simulink model "end_sem_mimuro_plot"  (R2023b)
settings: Solver=FixedStepAuto  StartTime=0.0  StopTime=20  FixedStep=0.001  RelTol=1e-3
undefined symbols (not defined in the file): simscape, X, Y, Z
libraries: sm_lib x108, nesl_utility x77, fl_lib x23, sdl_lib x5, sharedtransform x4
(part 6 of 6)

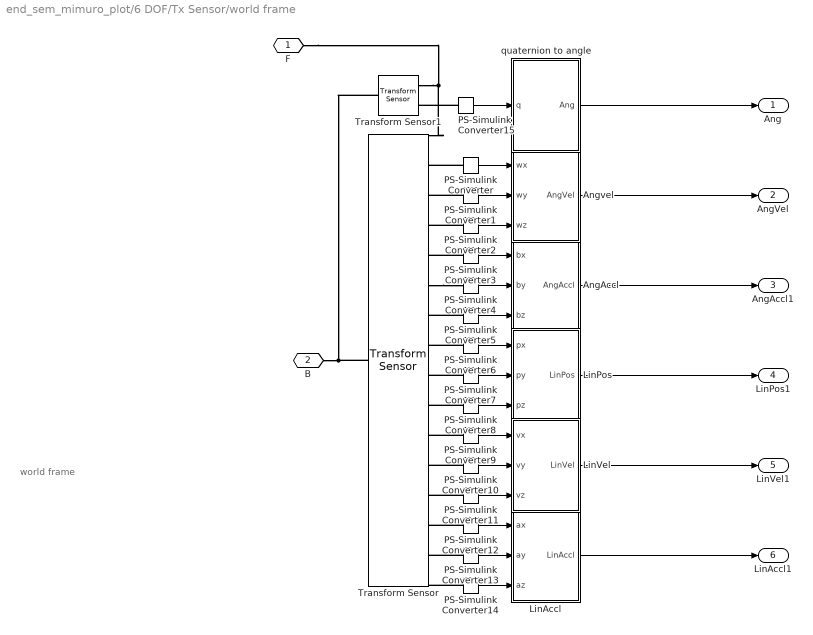
== system end_sem_mimuro_plot/6 DOF/Tx Sensor/world frame ==
  note: world frame
  AngAccl : Subsystem
  Angvel : Subsystem
  LinAccl : Subsystem
  LinPos : Subsystem
  LinVel : Subsystem
  PS-Simulink Converter{,1..15} (16 alike) : nesl_utility/PS-Simulink Converter  PhysicalDomain=network_engine_domain  SubClassName=ps_output  LeftPortType=input  RightPortType=output  PseudoPeriodic=off  Frequencies=[]  VectorFormat=1-D array  Unit=inherit  AffineConversion=off
  Transform Sensor1 : sm_lib/Frames and Transforms/Transform Sensor  MeasurementFrame=World  RotationSequence=XYX  SenseAngle=off  SenseAxis=off  SenseQ=on  SenseR=off  SenseRotationSequence=off  SenseOmegaX=off  SenseOmegaY=off  SenseOmegaZ=off  SenseOmega=off  SenseQDot=off  SenseRDot=off  SenseRotationSequenceDot=off  SenseAlphaX=off  SenseAlphaY=off  SenseAlphaZ=off  SenseAlpha=off  SenseQDDot=off  SenseRDDot=off  SenseX=off  SenseY=off  SenseZ=off  SenseXYZ=off  SenseRad=off  SenseAzim=off  SenseDist=off  SenseInc=off  SenseXDot=off  SenseYDot=off  SenseZDot=off  SenseXYZDot=off  SenseRadDot=off  SenseAzimDot=off  SenseDistDot=off  SenseIncDot=off  SenseXDDot=off  SenseYDDot=off  SenseZDDot=off  SenseXYZDDot=off  SenseRadDDot=off  SenseAzimDDot=off  SenseDistDDot=off  SenseIncDDot=off
  Transform Sensor : sm_lib/Frames and Transforms/Transform Sensor  MeasurementFrame=World  RotationSequence=XYX  SenseAngle=off  SenseAxis=off  SenseQ=off  SenseR=off  SenseRotationSequence=off  SenseOmegaX=on  SenseOmegaY=on  SenseOmegaZ=on  SenseOmega=off  SenseQDot=off  SenseRDot=off  SenseRotationSequenceDot=off  SenseAlphaX=on  SenseAlphaY=on  SenseAlphaZ=on  SenseAlpha=off  SenseQDDot=off  SenseRDDot=off  SenseX=on  SenseY=on  SenseZ=on  SenseXYZ=off  SenseRad=off  SenseAzim=off  SenseDist=off  SenseInc=off  SenseXDot=on  SenseYDot=on  SenseZDot=on  SenseXYZDot=off  SenseRadDot=off  SenseAzimDot=off  SenseDistDot=off  SenseIncDot=off  SenseXDDot=on  SenseYDDot=on  SenseZDDot=on  SenseXYZDDot=off  SenseRadDDot=off  SenseAzimDDot=off  SenseDistDDot=off  SenseIncDDot=off
  quaternion to angle : Subsystem
  F : PMIOPort  Side=Left
  B : PMIOPort  Port=2  Side=Left
  Ang : Outport
  AngVel : Outport  Port=2
  AngAccl1 : Outport  Port=3
  LinPos1 : Outport  Port=4
  LinVel1 : Outport  Port=5
  LinAccl1 : Outport  Port=6
  wires:
  PS-Simulink Converter6/1 -> LinPos/1(px)
  PS-Simulink Converter4/1 -> AngAccl/2(by)
  PS-Simulink Converter14/1 -> LinAccl/3(az)
  PS-Simulink Converter10/1 -> LinVel/2(vy)
  PS-Simulink Converter3/1 -> AngAccl/1(bx)
  PS-Simulink Converter11/1 -> LinVel/3(vz)
  PS-Simulink Converter2/1 -> Angvel/3(wz)
  PS-Simulink Converter9/1 -> LinVel/1(vx)
  PS-Simulink Converter12/1 -> LinAccl/1(ax)
  PS-Simulink Converter13/1 -> LinAccl/2(ay)
  PS-Simulink Converter8/1 -> LinPos/3(pz)
  PS-Simulink Converter1/1 -> Angvel/2(wy)
  LinVel/1(LinVel) -> LinVel1/1
  PS-Simulink Converter/1 -> Angvel/1(wx)
  PS-Simulink Converter5/1 -> AngAccl/3(bz)
  PS-Simulink Converter15/1 -> quaternion to angle/1(q)
  PS-Simulink Converter7/1 -> LinPos/2(py)
  LinPos/1(LinPos) -> LinPos1/1
  LinAccl/1(LinAccl) -> LinAccl1/1
  AngAccl/1(AngAccl) -> AngAccl1/1
  Angvel/1(AngVel) -> AngVel/1
  quaternion to angle/1(Ang) -> Ang/1
  connections:
  Transform Sensor1/RConn1 -- Transform Sensor/RConn1 -- F/RConn1
  PS-Simulink Converter/LConn1 -- Transform Sensor/RConn2
  PS-Simulink Converter1/LConn1 -- Transform Sensor/RConn3
  PS-Simulink Converter12/LConn1 -- Transform Sensor/RConn14
  PS-Simulink Converter3/LConn1 -- Transform Sensor/RConn5
  PS-Simulink Converter2/LConn1 -- Transform Sensor/RConn4
  PS-Simulink Converter14/LConn1 -- Transform Sensor/RConn16
  PS-Simulink Converter7/LConn1 -- Transform Sensor/RConn9
  Transform Sensor/RConn6 -- PS-Simulink Converter4/LConn1
  PS-Simulink Converter5/LConn1 -- Transform Sensor/RConn7
  PS-Simulink Converter8/LConn1 -- Transform Sensor/RConn10
  PS-Simulink Converter6/LConn1 -- Transform Sensor/RConn8
  PS-Simulink Converter15/LConn1 -- Transform Sensor1/RConn2
  PS-Simulink Converter9/LConn1 -- Transform Sensor/RConn11
  PS-Simulink Converter13/LConn1 -- Transform Sensor/RConn15
  PS-Simulink Converter10/LConn1 -- Transform Sensor/RConn12
  PS-Simulink Converter11/LConn1 -- Transform Sensor/RConn13
  B/RConn1 -- Transform Sensor/LConn1 -- Transform Sensor1/LConn1

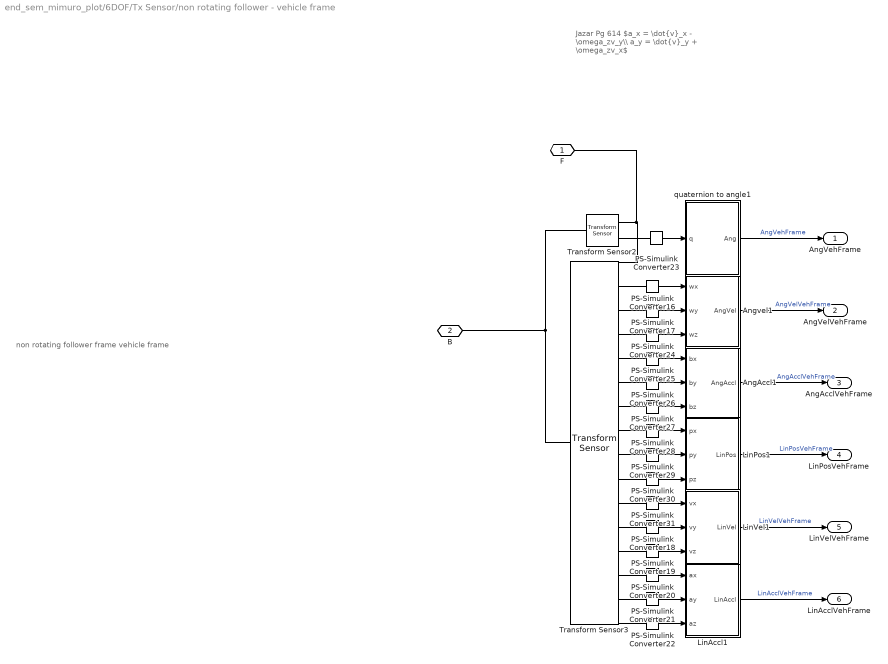
== system end_sem_mimuro_plot/6DOF/Tx Sensor/non rotating follower - vehicle frame ==
  note: non rotating follower frame
      | vehicle frame
  note: Jazar Pg 614
      | $a_x = \dot{v}_x - \omega_zv_y\\ a_y = \dot{v}_y + \omega_zv_x$
  AngAccl1 : Subsystem
  Angvel1 : Subsystem
  LinAccl1 : Subsystem
  LinPos1 : Subsystem
  LinVel1 : Subsystem
  PS-Simulink Converter{16..31} (16 alike) : nesl_utility/PS-Simulink Converter  PhysicalDomain=network_engine_domain  SubClassName=ps_output  LeftPortType=input  RightPortType=output  PseudoPeriodic=off  Frequencies=[]  VectorFormat=1-D array  Unit=inherit  AffineConversion=off
  Transform Sensor2 : sm_lib/Frames and Transforms/Transform Sensor  MeasurementFrame=NonRotatingFollower  RotationSequence=XYX  SenseAngle=off  SenseAxis=off  SenseQ=on  SenseR=off  SenseRotationSequence=off  SenseOmegaX=off  SenseOmegaY=off  SenseOmegaZ=off  SenseOmega=off  SenseQDot=off  SenseRDot=off  SenseRotationSequenceDot=off  SenseAlphaX=off  SenseAlphaY=off  SenseAlphaZ=off  SenseAlpha=off  SenseQDDot=off  SenseRDDot=off  SenseX=off  SenseY=off  SenseZ=off  SenseXYZ=off  SenseRad=off  SenseAzim=off  SenseDist=off  SenseInc=off  SenseXDot=off  SenseYDot=off  SenseZDot=off  SenseXYZDot=off  SenseRadDot=off  SenseAzimDot=off  SenseDistDot=off  SenseIncDot=off  SenseXDDot=off  SenseYDDot=off  SenseZDDot=off  SenseXYZDDot=off  SenseRadDDot=off  SenseAzimDDot=off  SenseDistDDot=off  SenseIncDDot=off
  Transform Sensor3 : sm_lib/Frames and Transforms/Transform Sensor  MeasurementFrame=NonRotatingFollower  RotationSequence=XYX  SenseAngle=off  SenseAxis=off  SenseQ=off  SenseR=off  SenseRotationSequence=off  SenseOmegaX=on  SenseOmegaY=on  SenseOmegaZ=on  SenseOmega=off  SenseQDot=off  SenseRDot=off  SenseRotationSequenceDot=off  SenseAlphaX=on  SenseAlphaY=on  SenseAlphaZ=on  SenseAlpha=off  SenseQDDot=off  SenseRDDot=off  SenseX=on  SenseY=on  SenseZ=on  SenseXYZ=off  SenseRad=off  SenseAzim=off  SenseDist=off  SenseInc=off  SenseXDot=on  SenseYDot=on  SenseZDot=on  SenseXYZDot=off  SenseRadDot=off  SenseAzimDot=off  SenseDistDot=off  SenseIncDot=off  SenseXDDot=on  SenseYDDot=on  SenseZDDot=on  SenseXYZDDot=off  SenseRadDDot=off  SenseAzimDDot=off  SenseDistDDot=off  SenseIncDDot=off
  quaternion to angle1 : Subsystem
  F : PMIOPort  Side=Left
  B : PMIOPort  Port=2  Side=Left
  AngVehFrame : Outport
  AngVelVehFrame : Outport  Port=2
  AngAcclVehFrame : Outport  Port=3
  LinPosVehFrame : Outport  Port=4
  LinVelVehFrame : Outport  Port=5
  LinAcclVehFrame : Outport  Port=6
  wires:
  PS-Simulink Converter16/1 -> Angvel1/1(wx)
  PS-Simulink Converter25/1 -> AngAccl1/1(bx)
  PS-Simulink Converter27/1 -> AngAccl1/3(bz)
  PS-Simulink Converter19/1 -> LinVel1/3(vz)
  quaternion to angle1/1(Ang) -> AngVehFrame/1  "AngVehFrame"
  PS-Simulink Converter20/1 -> LinAccl1/1(ax)
  Angvel1/1(AngVel) -> AngVelVehFrame/1  "AngVelVehFrame"
  PS-Simulink Converter31/1 -> LinVel1/1(vx)
  PS-Simulink Converter28/1 -> LinPos1/1(px)
  PS-Simulink Converter18/1 -> LinVel1/2(vy)
  PS-Simulink Converter30/1 -> LinPos1/3(pz)
  PS-Simulink Converter21/1 -> LinAccl1/2(ay)
  PS-Simulink Converter23/1 -> quaternion to angle1/1(q)
  PS-Simulink Converter22/1 -> LinAccl1/3(az)
  PS-Simulink Converter17/1 -> Angvel1/2(wy)
  PS-Simulink Converter24/1 -> Angvel1/3(wz)
  PS-Simulink Converter26/1 -> AngAccl1/2(by)
  PS-Simulink Converter29/1 -> LinPos1/2(py)
  LinVel1/1(LinVel) -> LinVelVehFrame/1  "LinVelVehFrame"
  AngAccl1/1(AngAccl) -> AngAcclVehFrame/1  "AngAcclVehFrame"
  LinPos1/1(LinPos) -> LinPosVehFrame/1  "LinPosVehFrame"
  LinAccl1/1(LinAccl) -> LinAcclVehFrame/1  "LinAcclVehFrame"
  connections:
  PS-Simulink Converter30/LConn1 -- Transform Sensor3/RConn10
  PS-Simulink Converter25/LConn1 -- Transform Sensor3/RConn5
  PS-Simulink Converter23/LConn1 -- Transform Sensor2/RConn2
  PS-Simulink Converter31/LConn1 -- Transform Sensor3/RConn11
  Transform Sensor2/LConn1 -- Transform Sensor3/LConn1 -- B/RConn1
  PS-Simulink Converter20/LConn1 -- Transform Sensor3/RConn14
  Transform Sensor2/RConn1 -- F/RConn1 -- Transform Sensor3/RConn1
  PS-Simulink Converter21/LConn1 -- Transform Sensor3/RConn15
  PS-Simulink Converter24/LConn1 -- Transform Sensor3/RConn4
  PS-Simulink Converter29/LConn1 -- Transform Sensor3/RConn9
  PS-Simulink Converter22/LConn1 -- Transform Sensor3/RConn16
  PS-Simulink Converter27/LConn1 -- Transform Sensor3/RConn7
  PS-Simulink Converter18/LConn1 -- Transform Sensor3/RConn12
  PS-Simulink Converter28/LConn1 -- Transform Sensor3/RConn8
  PS-Simulink Converter19/LConn1 -- Transform Sensor3/RConn13
  PS-Simulink Converter17/LConn1 -- Transform Sensor3/RConn3
  Transform Sensor3/RConn6 -- PS-Simulink Converter26/LConn1
  PS-Simulink Converter16/LConn1 -- Transform Sensor3/RConn2

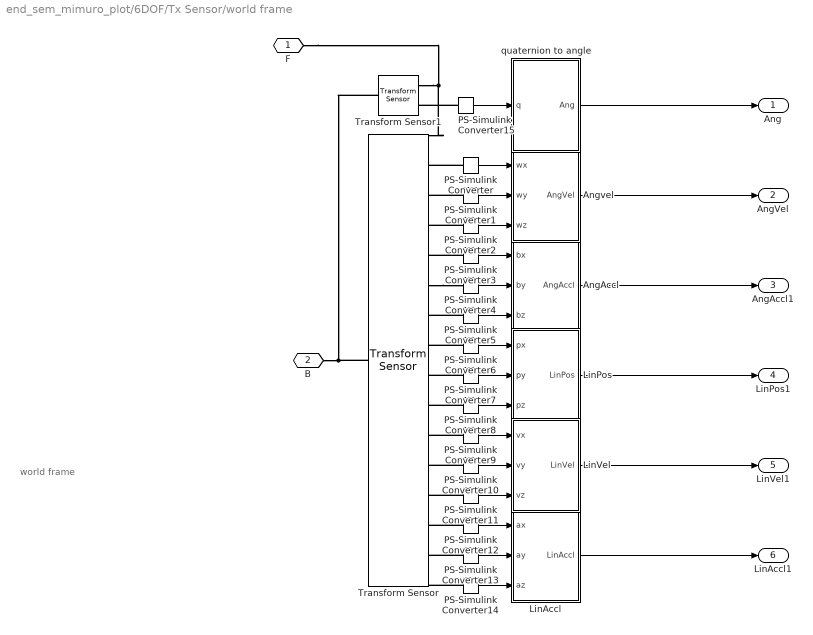
== system end_sem_mimuro_plot/6DOF/Tx Sensor/world frame ==
  note: world frame
  AngAccl : Subsystem
  Angvel : Subsystem
  LinAccl : Subsystem
  LinPos : Subsystem
  LinVel : Subsystem
  PS-Simulink Converter{,1..15} (16 alike) : nesl_utility/PS-Simulink Converter  PhysicalDomain=network_engine_domain  SubClassName=ps_output  LeftPortType=input  RightPortType=output  PseudoPeriodic=off  Frequencies=[]  VectorFormat=1-D array  Unit=inherit  AffineConversion=off
  Transform Sensor1 : sm_lib/Frames and Transforms/Transform Sensor  MeasurementFrame=World  RotationSequence=XYX  SenseAngle=off  SenseAxis=off  SenseQ=on  SenseR=off  SenseRotationSequence=off  SenseOmegaX=off  SenseOmegaY=off  SenseOmegaZ=off  SenseOmega=off  SenseQDot=off  SenseRDot=off  SenseRotationSequenceDot=off  SenseAlphaX=off  SenseAlphaY=off  SenseAlphaZ=off  SenseAlpha=off  SenseQDDot=off  SenseRDDot=off  SenseX=off  SenseY=off  SenseZ=off  SenseXYZ=off  SenseRad=off  SenseAzim=off  SenseDist=off  SenseInc=off  SenseXDot=off  SenseYDot=off  SenseZDot=off  SenseXYZDot=off  SenseRadDot=off  SenseAzimDot=off  SenseDistDot=off  SenseIncDot=off  SenseXDDot=off  SenseYDDot=off  SenseZDDot=off  SenseXYZDDot=off  SenseRadDDot=off  SenseAzimDDot=off  SenseDistDDot=off  SenseIncDDot=off
  Transform Sensor : sm_lib/Frames and Transforms/Transform Sensor  MeasurementFrame=World  RotationSequence=XYX  SenseAngle=off  SenseAxis=off  SenseQ=off  SenseR=off  SenseRotationSequence=off  SenseOmegaX=on  SenseOmegaY=on  SenseOmegaZ=on  SenseOmega=off  SenseQDot=off  SenseRDot=off  SenseRotationSequenceDot=off  SenseAlphaX=on  SenseAlphaY=on  SenseAlphaZ=on  SenseAlpha=off  SenseQDDot=off  SenseRDDot=off  SenseX=on  SenseY=on  SenseZ=on  SenseXYZ=off  SenseRad=off  SenseAzim=off  SenseDist=off  SenseInc=off  SenseXDot=on  SenseYDot=on  SenseZDot=on  SenseXYZDot=off  SenseRadDot=off  SenseAzimDot=off  SenseDistDot=off  SenseIncDot=off  SenseXDDot=on  SenseYDDot=on  SenseZDDot=on  SenseXYZDDot=off  SenseRadDDot=off  SenseAzimDDot=off  SenseDistDDot=off  SenseIncDDot=off
  quaternion to angle : Subsystem
  F : PMIOPort  Side=Left
  B : PMIOPort  Port=2  Side=Left
  Ang : Outport
  AngVel : Outport  Port=2
  AngAccl1 : Outport  Port=3
  LinPos1 : Outport  Port=4
  LinVel1 : Outport  Port=5
  LinAccl1 : Outport  Port=6
  wires:
  PS-Simulink Converter6/1 -> LinPos/1(px)
  PS-Simulink Converter4/1 -> AngAccl/2(by)
  PS-Simulink Converter14/1 -> LinAccl/3(az)
  PS-Simulink Converter10/1 -> LinVel/2(vy)
  PS-Simulink Converter3/1 -> AngAccl/1(bx)
  PS-Simulink Converter11/1 -> LinVel/3(vz)
  PS-Simulink Converter2/1 -> Angvel/3(wz)
  PS-Simulink Converter9/1 -> LinVel/1(vx)
  PS-Simulink Converter12/1 -> LinAccl/1(ax)
  PS-Simulink Converter13/1 -> LinAccl/2(ay)
  PS-Simulink Converter8/1 -> LinPos/3(pz)
  PS-Simulink Converter1/1 -> Angvel/2(wy)
  LinVel/1(LinVel) -> LinVel1/1
  PS-Simulink Converter/1 -> Angvel/1(wx)
  PS-Simulink Converter5/1 -> AngAccl/3(bz)
  PS-Simulink Converter15/1 -> quaternion to angle/1(q)
  PS-Simulink Converter7/1 -> LinPos/2(py)
  LinPos/1(LinPos) -> LinPos1/1
  LinAccl/1(LinAccl) -> LinAccl1/1
  AngAccl/1(AngAccl) -> AngAccl1/1
  Angvel/1(AngVel) -> AngVel/1
  quaternion to angle/1(Ang) -> Ang/1
  connections:
  Transform Sensor1/RConn1 -- Transform Sensor/RConn1 -- F/RConn1
  PS-Simulink Converter/LConn1 -- Transform Sensor/RConn2
  PS-Simulink Converter1/LConn1 -- Transform Sensor/RConn3
  PS-Simulink Converter12/LConn1 -- Transform Sensor/RConn14
  PS-Simulink Converter3/LConn1 -- Transform Sensor/RConn5
  PS-Simulink Converter2/LConn1 -- Transform Sensor/RConn4
  PS-Simulink Converter14/LConn1 -- Transform Sensor/RConn16
  PS-Simulink Converter7/LConn1 -- Transform Sensor/RConn9
  Transform Sensor/RConn6 -- PS-Simulink Converter4/LConn1
  PS-Simulink Converter5/LConn1 -- Transform Sensor/RConn7
  PS-Simulink Converter8/LConn1 -- Transform Sensor/RConn10
  PS-Simulink Converter6/LConn1 -- Transform Sensor/RConn8
  PS-Simulink Converter15/LConn1 -- Transform Sensor1/RConn2
  PS-Simulink Converter9/LConn1 -- Transform Sensor/RConn11
  PS-Simulink Converter13/LConn1 -- Transform Sensor/RConn15
  PS-Simulink Converter10/LConn1 -- Transform Sensor/RConn12
  PS-Simulink Converter11/LConn1 -- Transform Sensor/RConn13
  B/RConn1 -- Transform Sensor/LConn1 -- Transform Sensor1/LConn1

== system end_sem_mimuro_plot/6 DOF/Tx Sensor/non rotating follower - vehicle frame/AngAccl1 ==
  bx : Inport
  by : Inport  Port=2
  bz : Inport  Port=3
  bus creator4 : BusCreator  Inputs=3
  AngAccl : Outport
  wires:
  bx/1 -> bus creator4/1  "bx"
  by/1 -> bus creator4/2  "by"
  bz/1 -> bus creator4/3  "bz"
  bus creator4/1 -> AngAccl/1  "AngAcclVehFrame"

== system end_sem_mimuro_plot/6 DOF/Tx Sensor/non rotating follower - vehicle frame/Angvel1 ==
  wx : Inport
  wy : Inport  Port=2
  wz : Inport  Port=3
  bus creator4 : BusCreator  Inputs=3
  AngVel : Outport
  wires:
  bus creator4/1 -> AngVel/1  "AngVelVehFrame"
  wz/1 -> bus creator4/3  "wz"
  wy/1 -> bus creator4/2  "wy"
  wx/1 -> bus creator4/1  "wx"

== system end_sem_mimuro_plot/6 DOF/Tx Sensor/non rotating follower - vehicle frame/LinAccl1 ==
  ax : Inport
  ay : Inport  Port=2
  az : Inport  Port=3
  bus creator2 : BusCreator  Inputs=3
  LinAccl : Outport
  wires:
  bus creator2/1 -> LinAccl/1  "LinAcclVehFrame"
  az/1 -> bus creator2/3  "az"
  ax/1 -> bus creator2/1  "ax"
  ay/1 -> bus creator2/2  "ay"

== system end_sem_mimuro_plot/6 DOF/Tx Sensor/non rotating follower - vehicle frame/LinPos1 ==
  px : Inport
  py : Inport  Port=2
  pz : Inport  Port=3
  bus creator : BusCreator  Inputs=3
  LinPos : Outport
  wires:
  bus creator/1 -> LinPos/1  "LinPosVehFrame"
  px/1 -> bus creator/1  "px"
  pz/1 -> bus creator/3  "pz"
  py/1 -> bus creator/2  "py"

== system end_sem_mimuro_plot/6 DOF/Tx Sensor/non rotating follower - vehicle frame/LinVel1 ==
  vx : Inport
  vy : Inport  Port=2
  vz : Inport  Port=3
  bus creator1 : BusCreator  Inputs=3
  LinVel : Outport
  wires:
  vz/1 -> bus creator1/3  "vz"
  vy/1 -> bus creator1/2  "vy"
  vx/1 -> bus creator1/1  "vx"
  bus creator1/1 -> LinVel/1  "LinVelVehFrame"

== system end_sem_mimuro_plot/6 DOF/Tx Sensor/non rotating follower - vehicle frame/quaternion to angle1 ==
  q : Inport
  Quaternions to Rotation Angles : sharedtransform/Quaternions to Rotation Angles  rotationOrder=ZYX  aMode=aMode
  Selector : Selector  InputPortWidth=3  IndexOptions=Index vector (dialog)  Indices=3  OutputSizes=1
  Selector1 : Selector  InputPortWidth=3  IndexOptions=Index vector (dialog)  Indices=2  OutputSizes=1
  Selector2 : Selector  InputPortWidth=3  IndexOptions=Index vector (dialog)  Indices=1  OutputSizes=1
  bus creator3 : BusCreator  Inputs=3
  Ang : Outport
  wires:
  Quaternions to Rotation Angles/1 -> Selector1/1, Selector2/1, Selector/1
  Selector1/1 -> bus creator3/2  "ry"
  bus creator3/1 -> Ang/1  "AngVehFrame"
  Selector2/1 -> bus creator3/3  "rz"
  Selector/1 -> bus creator3/1  "rx"
  q/1 -> Quaternions to Rotation Angles/1

== system end_sem_mimuro_plot/6 DOF/Tx Sensor/world frame/AngAccl ==
  bx : Inport
  by : Inport  Port=2
  bz : Inport  Port=3
  bus creator4 : BusCreator  Inputs=3
  AngAccl : Outport
  wires:
  bus creator4/1 -> AngAccl/1  "AngAccl"
  bz/1 -> bus creator4/3  "bz"
  by/1 -> bus creator4/2  "by"
  bx/1 -> bus creator4/1  "bx"

== system end_sem_mimuro_plot/6 DOF/Tx Sensor/world frame/Angvel ==
  wx : Inport
  wy : Inport  Port=2
  wz : Inport  Port=3
  bus creator4 : BusCreator  Inputs=3
  AngVel : Outport
  wires:
  wx/1 -> bus creator4/1  "wx"
  wy/1 -> bus creator4/2  "wy"
  wz/1 -> bus creator4/3  "wz"
  bus creator4/1 -> AngVel/1  "AngVel"

== system end_sem_mimuro_plot/6 DOF/Tx Sensor/world frame/LinAccl ==
  ax : Inport
  ay : Inport  Port=2
  az : Inport  Port=3
  bus creator2 : BusCreator  Inputs=3
  LinAccl : Outport
  wires:
  ay/1 -> bus creator2/2  "ay"
  ax/1 -> bus creator2/1  "ax"
  az/1 -> bus creator2/3  "az"
  bus creator2/1 -> LinAccl/1  "LinAccl"

== system end_sem_mimuro_plot/6 DOF/Tx Sensor/world frame/LinPos ==
  px : Inport
  py : Inport  Port=2
  pz : Inport  Port=3
  bus creator : BusCreator  Inputs=3
  LinPos : Outport
  wires:
  py/1 -> bus creator/2  "py"
  pz/1 -> bus creator/3  "pz"
  px/1 -> bus creator/1  "px"
  bus creator/1 -> LinPos/1  "LinPos"

== system end_sem_mimuro_plot/6 DOF/Tx Sensor/world frame/LinVel ==
  vx : Inport
  vy : Inport  Port=2
  vz : Inport  Port=3
  bus creator1 : BusCreator  Inputs=3
  LinVel : Outport
  wires:
  bus creator1/1 -> LinVel/1  "LinVel"
  vx/1 -> bus creator1/1  "vx"
  vy/1 -> bus creator1/2  "vy"
  vz/1 -> bus creator1/3  "vz"

== system end_sem_mimuro_plot/6 DOF/Tx Sensor/world frame/quaternion to angle ==
  q : Inport
  Quaternions to Rotation Angles : sharedtransform/Quaternions to Rotation Angles  rotationOrder=ZYX  aMode=aMode
  Selector : Selector  InputPortWidth=3  IndexOptions=Index vector (dialog)  Indices=3  OutputSizes=1
  Selector1 : Selector  InputPortWidth=3  IndexOptions=Index vector (dialog)  Indices=2  OutputSizes=1
  Selector2 : Selector  InputPortWidth=3  IndexOptions=Index vector (dialog)  Indices=1  OutputSizes=1
  bus creator3 : BusCreator  Inputs=3
  Ang : Outport
  wires:
  q/1 -> Quaternions to Rotation Angles/1
  Selector/1 -> bus creator3/1  "rx"
  Selector2/1 -> bus creator3/3  "rz"
  bus creator3/1 -> Ang/1  "Ang"
  Selector1/1 -> bus creator3/2  "ry"
  Quaternions to Rotation Angles/1 -> Selector/1, Selector2/1, Selector1/1

== system end_sem_mimuro_plot/6DOF/Tx Sensor/non rotating follower - vehicle frame/AngAccl1 ==
  bx : Inport
  by : Inport  Port=2
  bz : Inport  Port=3
  bus creator4 : BusCreator  Inputs=3
  AngAccl : Outport
  wires:
  bx/1 -> bus creator4/1  "bx"
  by/1 -> bus creator4/2  "by"
  bz/1 -> bus creator4/3  "bz"
  bus creator4/1 -> AngAccl/1  "AngAcclVehFrame"

== system end_sem_mimuro_plot/6DOF/Tx Sensor/non rotating follower - vehicle frame/Angvel1 ==
  wx : Inport
  wy : Inport  Port=2
  wz : Inport  Port=3
  bus creator4 : BusCreator  Inputs=3
  AngVel : Outport
  wires:
  bus creator4/1 -> AngVel/1  "AngVelVehFrame"
  wz/1 -> bus creator4/3  "wz"
  wy/1 -> bus creator4/2  "wy"
  wx/1 -> bus creator4/1  "wx"

== system end_sem_mimuro_plot/6DOF/Tx Sensor/non rotating follower - vehicle frame/LinAccl1 ==
  ax : Inport
  ay : Inport  Port=2
  az : Inport  Port=3
  bus creator2 : BusCreator  Inputs=3
  LinAccl : Outport
  wires:
  bus creator2/1 -> LinAccl/1  "LinAcclVehFrame"
  az/1 -> bus creator2/3  "az"
  ax/1 -> bus creator2/1  "ax"
  ay/1 -> bus creator2/2  "ay"

== system end_sem_mimuro_plot/6DOF/Tx Sensor/non rotating follower - vehicle frame/LinPos1 ==
  px : Inport
  py : Inport  Port=2
  pz : Inport  Port=3
  bus creator : BusCreator  Inputs=3
  LinPos : Outport
  wires:
  bus creator/1 -> LinPos/1  "LinPosVehFrame"
  px/1 -> bus creator/1  "px"
  pz/1 -> bus creator/3  "pz"
  py/1 -> bus creator/2  "py"

== system end_sem_mimuro_plot/6DOF/Tx Sensor/non rotating follower - vehicle frame/LinVel1 ==
  vx : Inport
  vy : Inport  Port=2
  vz : Inport  Port=3
  bus creator1 : BusCreator  Inputs=3
  LinVel : Outport
  wires:
  vz/1 -> bus creator1/3  "vz"
  vy/1 -> bus creator1/2  "vy"
  vx/1 -> bus creator1/1  "vx"
  bus creator1/1 -> LinVel/1  "LinVelVehFrame"

== system end_sem_mimuro_plot/6DOF/Tx Sensor/non rotating follower - vehicle frame/quaternion to angle1 ==
  q : Inport
  Quaternions to Rotation Angles : sharedtransform/Quaternions to Rotation Angles  rotationOrder=ZYX  aMode=aMode
  Selector : Selector  InputPortWidth=3  IndexOptions=Index vector (dialog)  Indices=3  OutputSizes=1
  Selector1 : Selector  InputPortWidth=3  IndexOptions=Index vector (dialog)  Indices=2  OutputSizes=1
  Selector2 : Selector  InputPortWidth=3  IndexOptions=Index vector (dialog)  Indices=1  OutputSizes=1
  bus creator3 : BusCreator  Inputs=3
  Ang : Outport
  wires:
  Quaternions to Rotation Angles/1 -> Selector1/1, Selector2/1, Selector/1
  Selector1/1 -> bus creator3/2  "ry"
  bus creator3/1 -> Ang/1  "AngVehFrame"
  Selector2/1 -> bus creator3/3  "rz"
  Selector/1 -> bus creator3/1  "rx"
  q/1 -> Quaternions to Rotation Angles/1

== system end_sem_mimuro_plot/6DOF/Tx Sensor/world frame/AngAccl ==
  bx : Inport
  by : Inport  Port=2
  bz : Inport  Port=3
  bus creator4 : BusCreator  Inputs=3
  AngAccl : Outport
  wires:
  bus creator4/1 -> AngAccl/1  "AngAccl"
  bz/1 -> bus creator4/3  "bz"
  by/1 -> bus creator4/2  "by"
  bx/1 -> bus creator4/1  "bx"

== system end_sem_mimuro_plot/6DOF/Tx Sensor/world frame/Angvel ==
  wx : Inport
  wy : Inport  Port=2
  wz : Inport  Port=3
  bus creator4 : BusCreator  Inputs=3
  AngVel : Outport
  wires:
  wx/1 -> bus creator4/1  "wx"
  wy/1 -> bus creator4/2  "wy"
  wz/1 -> bus creator4/3  "wz"
  bus creator4/1 -> AngVel/1  "AngVel"

== system end_sem_mimuro_plot/6DOF/Tx Sensor/world frame/LinAccl ==
  ax : Inport
  ay : Inport  Port=2
  az : Inport  Port=3
  bus creator2 : BusCreator  Inputs=3
  LinAccl : Outport
  wires:
  ay/1 -> bus creator2/2  "ay"
  ax/1 -> bus creator2/1  "ax"
  az/1 -> bus creator2/3  "az"
  bus creator2/1 -> LinAccl/1  "LinAccl"

== system end_sem_mimuro_plot/6DOF/Tx Sensor/world frame/LinPos ==
  px : Inport
  py : Inport  Port=2
  pz : Inport  Port=3
  bus creator : BusCreator  Inputs=3
  LinPos : Outport
  wires:
  py/1 -> bus creator/2  "py"
  pz/1 -> bus creator/3  "pz"
  px/1 -> bus creator/1  "px"
  bus creator/1 -> LinPos/1  "LinPos"

== system end_sem_mimuro_plot/6DOF/Tx Sensor/world frame/LinVel ==
  vx : Inport
  vy : Inport  Port=2
  vz : Inport  Port=3
  bus creator1 : BusCreator  Inputs=3
  LinVel : Outport
  wires:
  bus creator1/1 -> LinVel/1  "LinVel"
  vx/1 -> bus creator1/1  "vx"
  vy/1 -> bus creator1/2  "vy"
  vz/1 -> bus creator1/3  "vz"

== system end_sem_mimuro_plot/6DOF/Tx Sensor/world frame/quaternion to angle ==
  q : Inport
  Quaternions to Rotation Angles : sharedtransform/Quaternions to Rotation Angles  rotationOrder=ZYX  aMode=aMode
  Selector : Selector  InputPortWidth=3  IndexOptions=Index vector (dialog)  Indices=3  OutputSizes=1
  Selector1 : Selector  InputPortWidth=3  IndexOptions=Index vector (dialog)  Indices=2  OutputSizes=1
  Selector2 : Selector  InputPortWidth=3  IndexOptions=Index vector (dialog)  Indices=1  OutputSizes=1
  bus creator3 : BusCreator  Inputs=3
  Ang : Outport
  wires:
  q/1 -> Quaternions to Rotation Angles/1
  Selector/1 -> bus creator3/1  "rx"
  Selector2/1 -> bus creator3/3  "rz"
  bus creator3/1 -> Ang/1  "Ang"
  Selector1/1 -> bus creator3/2  "ry"
  Quaternions to Rotation Angles/1 -> Selector/1, Selector2/1, Selector1/1
